simulink model "trenl"  (R2022a)
settings: Solver=FixedStepDiscrete  StartTime=0.0  StopTime=10.0  FixedStep=0.001  RelTol=1e-3
values from neighbouring files (symbols this model uses):
  to = round(rand*100)    [test_model.m]
  Ts = 0.001    [test_model.m]
undefined symbols (not defined in the file or in its folder): Am, NP, R
libraries: commanapbnd3 x2
settings Model: Creator=sssss  LastModifiedBy=Веточка

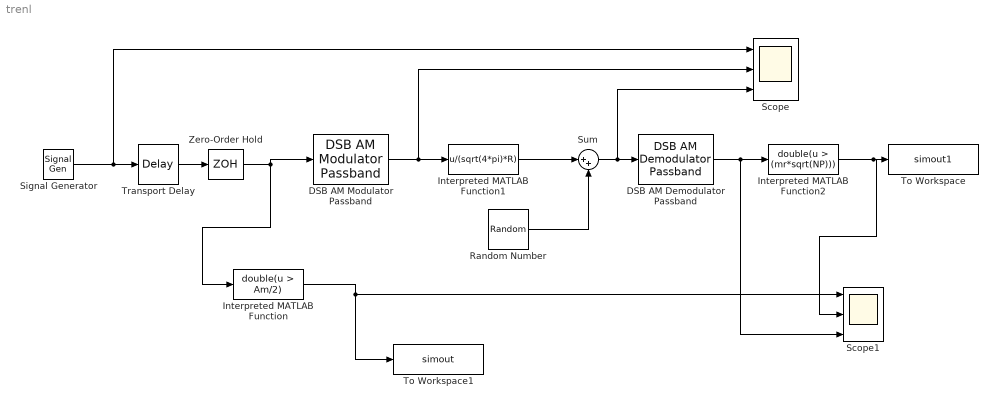
== system trenl ==
  DSB AM Demodulator Passband : commanapbnd3/DSB AM Demodulator Passband  Fc=600  Ph=0  method=Butterworth  n=4  cf=100  Rp=0.1  Rs=50  Offset=0
      settings: SourceProductBaseCode=CM
  DSB AM Modulator Passband : commanapbnd3/DSB AM Modulator Passband  Fc=600  Ph=0  Offset=0
      settings: SourceProductBaseCode=CM
  Interpreted MATLAB Function : MATLABFcn  MATLABFcn=double(u > Am/2)  Output1D=off
  Interpreted MATLAB Function1 : MATLABFcn  MATLABFcn=u/(sqrt(4*pi)*R)  Output1D=off
  Interpreted MATLAB Function2 : MATLABFcn  MATLABFcn=double(u > (mr*sqrt(NP)))  Output1D=off
  Random Number : RandomNumber  Variance=NP  Seed=to  SampleTime=Ts
  Scope : Scope  NumInputPorts=3
  Scope1 : Scope  NumInputPorts=3
  Signal Generator : SignalGenerator  Amplitude=Am  Frequency=20
  Sum : Sum  Inputs=|++
  To Workspace : ToWorkspace  VariableName=simout1  SampleTime=-1
      settings: Save2DSignal=2-D array (concatenate along first dimension)
  To Workspace1 : ToWorkspace  VariableName=simout  SampleTime=-1
      settings: Save2DSignal=2-D array (concatenate along first dimension)
  Transport Delay : TransportDelay  DelayTime=4.5  BufferSize=10240
  Zero-Order Hold : ZeroOrderHold  SampleTime=Ts
  wires:
  Transport Delay/1 -> Zero-Order Hold/1
  Interpreted MATLAB Function/1 -> To Workspace1/1, Scope1/1
  Interpreted MATLAB Function1/1 -> Sum/1
  DSB AM Modulator Passband/1 -> Scope/2, Interpreted MATLAB Function1/1
  Random Number/1 -> Sum/2
  Sum/1 -> DSB AM Demodulator Passband/1, Scope/3
  DSB AM Demodulator Passband/1 -> Scope1/3, Interpreted MATLAB Function2/1
  Interpreted MATLAB Function2/1 -> Scope1/2, To Workspace/1
  Zero-Order Hold/1 -> Interpreted MATLAB Function/1, DSB AM Modulator Passband/1
  Signal Generator/1 -> Transport Delay/1, Scope/1
